simulink model "SLX1"  (R2019b)
settings: Solver=VariableStepAuto  StartTime=0.0  StopTime=500  MaxStep=1  RelTol=1e-3
undefined symbols (not defined in the file or in its folder): k0, k10, k12, k21
settings Model: OrderedModelArguments=off  Creator=Dgy  LastModifiedBy=Dgy
settings SolverCC: InitialStep=1
settings OptimizationCC: LifeSpan=inf
settings DebuggingCC: ArithmeticOperatorsInVariantConditions=warning
settings SFSimCC: CustomCodeUndefinedFunction=UseInterfaceOnly
settings CodeAppCC: StateflowObjectComments=on

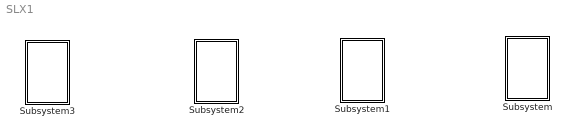
== system SLX1 ==
  Subsystem : Subsystem
      settings: AttributesFormatString=二室模型口服给药
  Subsystem1 : Subsystem
      settings: AttributesFormatString=二室模型注射给药
  Subsystem2 : Subsystem
      settings: AttributesFormatString=一室模型口服给药
  Subsystem3 : Subsystem
      settings: AttributesFormatString=一室模型注射给药

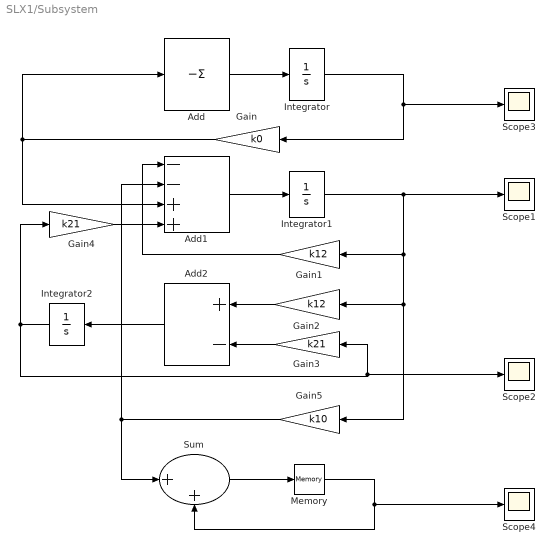
== system SLX1/Subsystem ==
  Add : Sum  Inputs=-
      settings: AttributesFormatString=吸收
      mask Display: image('$imagefile'); % Use "Edit Image" on toolstrip to change.
  Add1 : Sum  Inputs=--++
      settings: AttributesFormatString=中央室(一室)
      mask Display: image('$imagefile'); % Use "Edit Image" on toolstrip to change.
  Add2 : Sum  Inputs=+-
      settings: AttributesFormatString=周边室(二室)
      mask Display: image('$imagefile'); % Use "Edit Image" on toolstrip to change.
  Gain : Gain  Gain=k0
  Gain1 : Gain  Gain=k12
  Gain2 : Gain  Gain=k12
  Gain3 : Gain  Gain=k21
  Gain4 : Gain  Gain=k21
  Gain5 : Gain  Gain=k10
  Integrator : Integrator  InitialCondition=100
  Integrator1 : Integrator
  Integrator2 : Integrator
  Memory : Memory
  Scope{1..4} (4 alike) : Scope
      Scope1 settings: AttributesFormatString=血液系统
      Scope2 settings: AttributesFormatString=脑、肺、肝
      Scope3 settings: AttributesFormatString=胃
      Scope4 settings: AttributesFormatString=肾、小肠、大肠
  Sum : Sum  Inputs=|++
      settings: AttributesFormatString=排泄、代谢
      mask Display: image('D:\simulinkPKPD\kidney.jpg'); % Use "Edit Image" on toolstrip to change.
  wires:
  Integrator2/1 -> Scope2/1, Gain3/1, Gain4/1
  Add/1 -> Integrator/1
  Gain/1 -> Add1/3, Add/1
  Gain1/1 -> Add1/1
  Gain3/1 -> Add2/2
  Integrator1/1 -> Gain5/1, Gain2/1, Gain1/1, Scope1/1
  Add1/1 -> Integrator1/1
  Sum/1 -> Memory/1
  Gain5/1 -> Add1/2, Sum/1
  Gain2/1 -> Add2/1
  Gain4/1 -> Add1/4
  Integrator/1 -> Gain/1, Scope3/1
  Add2/1 -> Integrator2/1
  Memory/1 -> Sum/2, Scope4/1

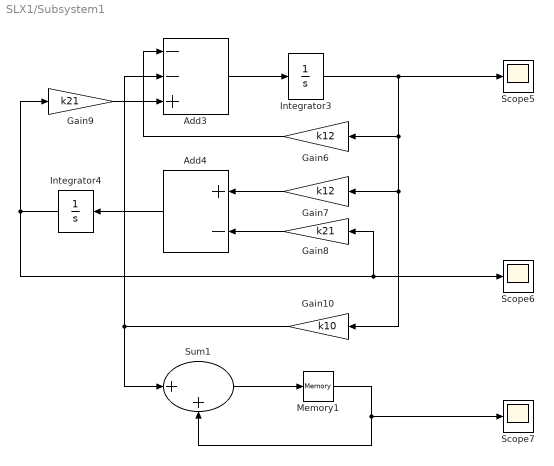
== system SLX1/Subsystem1 ==
  Add3 : Sum  Inputs=--+
      mask Display: image('$imagefile'); % Use "Edit Image" on toolstrip to change.
  Add4 : Sum  Inputs=+-
      mask Display: image('$imagefile'); % Use "Edit Image" on toolstrip to change.
  Gain10 : Gain  Gain=k10
  Gain6 : Gain  Gain=k12
  Gain7 : Gain  Gain=k12
  Gain8 : Gain  Gain=k21
  Gain9 : Gain  Gain=k21
  Integrator3 : Integrator  InitialCondition=100
  Integrator4 : Integrator
  Memory1 : Memory
  Scope5 : Scope
  Scope6 : Scope
  Scope7 : Scope
  Sum1 : Sum  Inputs=|++
      settings: AttributesFormatString=排泄、代谢
      mask Display: image('D:\simulinkPKPD\kidney.jpg'); % Use "Edit Image" on toolstrip to change.
  wires:
  Gain10/1 -> Add3/2, Sum1/1
  Sum1/1 -> Memory1/1
  Integrator3/1 -> Gain6/1, Gain10/1, Gain7/1, Scope5/1
  Gain7/1 -> Add4/1
  Gain6/1 -> Add3/1
  Add3/1 -> Integrator3/1
  Add4/1 -> Integrator4/1
  Integrator4/1 -> Gain9/1, Scope6/1, Gain8/1
  Memory1/1 -> Scope7/1, Sum1/2
  Gain9/1 -> Add3/3
  Gain8/1 -> Add4/2

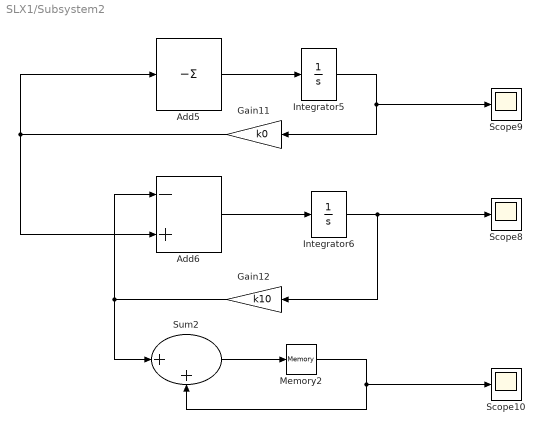
== system SLX1/Subsystem2 ==
  Add5 : Sum  Inputs=-
      mask Display: image('$imagefile'); % Use "Edit Image" on toolstrip to change.
  Add6 : Sum  Inputs=-+
      mask Display: image('$imagefile'); % Use "Edit Image" on toolstrip to change.
  Gain11 : Gain  Gain=k0
  Gain12 : Gain  Gain=k10
  Integrator5 : Integrator  InitialCondition=100
  Integrator6 : Integrator
  Memory2 : Memory
  Scope10 : Scope
      settings: AttributesFormatString=肾、小肠、大肠
  Scope8 : Scope
  Scope9 : Scope
  Sum2 : Sum  Inputs=|++
      settings: AttributesFormatString=排泄、代谢
      mask Display: image('D:\simulinkPKPD\kidney.jpg'); % Use "Edit Image" on toolstrip to change.
  wires:
  Gain11/1 -> Add5/1, Add6/2
  Sum2/1 -> Memory2/1
  Memory2/1 -> Sum2/2, Scope10/1
  Integrator5/1 -> Gain11/1, Scope9/1
  Add6/1 -> Integrator6/1
  Integrator6/1 -> Gain12/1, Scope8/1
  Add5/1 -> Integrator5/1
  Gain12/1 -> Sum2/1, Add6/1

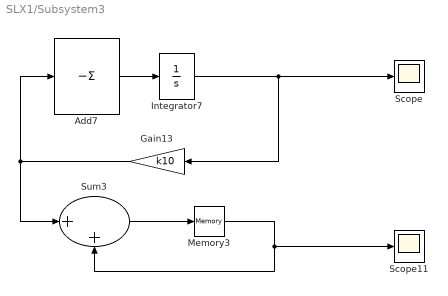
== system SLX1/Subsystem3 ==
  Add7 : Sum  Inputs=-
      mask Display: image('$imagefile'); % Use "Edit Image" on toolstrip to change.
  Gain13 : Gain  Gain=k10
  Integrator7 : Integrator  InitialCondition=100
  Memory3 : Memory
  Scope : Scope
  Scope11 : Scope
      settings: AttributesFormatString=肾、小肠、大肠
  Sum3 : Sum  Inputs=|++
      settings: AttributesFormatString=排泄、代谢
      mask Display: image('D:\simulinkPKPD\kidney.jpg'); % Use "Edit Image" on toolstrip to change.
  wires:
  Gain13/1 -> Add7/1, Sum3/1
  Add7/1 -> Integrator7/1
  Integrator7/1 -> Gain13/1, Scope/1
  Memory3/1 -> Sum3/2, Scope11/1
  Sum3/1 -> Memory3/1
